simulink model "controlScheme_height"  (R2019b)
settings: Solver=FixedStepDiscrete  StartTime=0.0  StopTime=Inf  FixedStep=1/30  RelTol=1e-3
InitFcn:
  | tb = twinbeam('147.32.86.177', 30000);
  | gen = generator('147.32.86.177', 30001);
  | img = tb.get();
  | f = figure(25)
  | imshow(img);
  | [x_t, y_t] = ginput(1);
  | 
  | tb.tracker_init([y_t, x_t]);
  | 
  | 
  | delete(tb)
  | delete(gen)
  | pause(4)
  | close(f)
model workspace (MAT data in the model file):
  NumberOfBeads = Simulink.Parameter
  NumberOfBeads.Value = 1
  NumberOfBeads.DataType = 'auto'
  NumberOfBeads.Dimensions = [1 1]
undefined symbols (not defined in the file): DiscIntNeverNeededParam, H, Joystick, Standard_Devices, TCP_Protocol
libraries: sldrtlib x5, simulink x1
settings Model: SimulationMode=accelerator  EnablePacing=on  ParameterArgumentNames=NumberOfBeads  OrderedModelArguments=off  Creator=marti  LastModifiedBy=marti
settings SolverCC: MinimalZcImpactIntegration=on
settings DebuggingCC: ReadBeforeWriteMsg=DisableAll  WriteAfterWriteMsg=DisableAll  WriteAfterReadMsg=DisableAll  MultiTaskDSMMsg=none
settings ModelReferenceCC: UpdateModelReferenceTargets=IfOutOfDate
settings SFSimCC: SFSimEcho=off
settings RTWCC: Description=Simulink Desktop Real-Time  SystemTargetFile=sldrt.tlc  TemplateMakefile=sldrt.tmf  RTWCompilerOptimization=on
settings CodeAppCC: MaxIdLength=95
settings SimulinkDesktopRealTimeCC: TargetPreCompLibLocation=C:\Program Files\MATLAB\R2020a\toolbox\sldrt\lib\win64

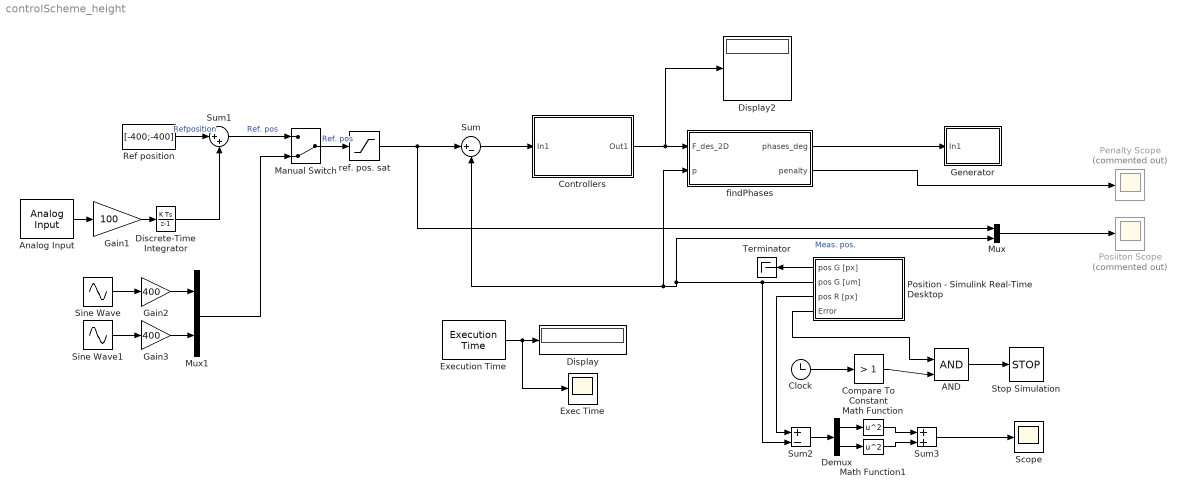
== system controlScheme_height ==
  AND : Logic  IconShape=distinctive  AllPortsSameDT=off  OutDataTypeStr=boolean
  Analog Input : sldrtlib/Analog Input  SampleTime=0.1  MaxMissedTicks=10  ShowMissedTicks=off  YieldWhenWaiting=off  DrvName=Standard_Devices/Joystick  DrvAddress=1  DrvOptions=zeros(1,0)  Channels=[1:2]  RangeMode=1  VoltRange=1  DataType=1
      settings: AttributesFormatString=Joystick [1]
  Clock : Clock
  Compare To Constant : simulink/Logic and Bit Operations/Compare To Constant  relop=>  const=1  OutDataTypeStr=boolean
  Controllers : Subsystem  mask{P_const=300e-14, F_max=30e-11}
      mask prompts: P_const "P constant"; F_max "F max"
  Demux : Demux  Outputs=2
  Discrete-Time Integrator : DiscreteIntegrator  gainval=1  SampleTime=-1  ICPrevOutput=DiscIntNeverNeededParam  ICPrevScaledInput=DiscIntNeverNeededParam
  Display : Display
  Display2 : Display
  Exec Time : Scope
  Execution Time : sldrtlib/Target Profiling/Execution Time  ShowTaskTimes=off
      settings: SourceProductBaseCode=WT
  Gain1 : Gain  Gain=100
  Gain2 : Gain  Gain=400
  Gain3 : Gain  Gain=400
  Generator : Subsystem
  Manual Switch : ManualSwitch  CurrentSetting=0
  Math Function : Math  Operator=square  SaturateOnIntegerOverflow=on
  Math Function1 : Math  Operator=square  SaturateOnIntegerOverflow=on
  Mux : Mux  Inputs=2
  Mux1 : Mux  Inputs=2
  Penalty Scope : Scope  Commented=on
  Posiiton Scope : Scope  Commented=on
  Position - Simulink Real-Time Desktop : Subsystem  VariantControl=(default)
  Ref position : Constant  Value=[-400;-400]
  Scope : Scope
  Sine Wave : Sin  Frequency=2*pi/40  SampleTime=0
  Sine Wave1 : Sin  Frequency=2*pi/20  Phase=-pi  SampleTime=0
  Stop Simulation : Stop
  Sum : Sum  Inputs=|+-
  Sum1 : Sum  Inputs=|++
  Sum2 : Sum  Inputs=+-
  Sum3 : Sum
  Terminator : Terminator
  findPhases : MATLAB Function  TreatAsAtomicUnit=on
  ref. pos. sat : Saturate  UpperLimit=600  LowerLimit=-600
  wires:
  Manual Switch/1 -> ref. pos. sat/1  "Ref. pos"
  Sum/1 -> Controllers/1(In1)
  Controllers/1(Out1) -> findPhases/1(F_des_2D), Display2/1
  Position - Simulink Real-Time Desktop/2(pos G [um]) -> Sum2/2, findPhases/2(p), Sum/2, Mux/2  "Meas. pos."
  Execution Time/1 -> Exec Time/1, Display/1
  findPhases/1(phases_deg) -> Generator/1(In1)
  findPhases/2(penalty) -> Penalty Scope/1
  AND/1 -> Stop Simulation/1
  Clock/1 -> Compare To Constant/1
  Compare To Constant/1 -> AND/2
  Position - Simulink Real-Time Desktop/4(Error) -> AND/1
  Mux/1 -> Posiiton Scope/1
  Analog Input/1 -> Gain1/1
  Ref position/1 -> Sum1/1  "Refposition"
  Discrete-Time Integrator/1 -> Sum1/2
  Gain1/1 -> Discrete-Time Integrator/1
  Sum1/1 -> Manual Switch/1  "Ref. pos"
  Sine Wave/1 -> Gain2/1
  Sine Wave1/1 -> Gain3/1
  Gain2/1 -> Mux1/1
  Gain3/1 -> Mux1/2
  Mux1/1 -> Manual Switch/2
  Position - Simulink Real-Time Desktop/1(pos G [px]) -> Terminator/1
  ref. pos. sat/1 -> Sum/1, Mux/1
  Position - Simulink Real-Time Desktop/3(pos R [px]) -> Sum2/1
  Sum2/1 -> Demux/1
  Demux/1 -> Math Function/1
  Demux/2 -> Math Function1/1
  Math Function/1 -> Sum3/1
  Math Function1/1 -> Sum3/2
  Sum3/1 -> Scope/1

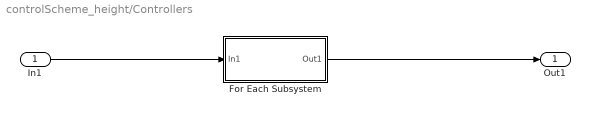
== system controlScheme_height/Controllers ==
  In1 : Inport
  For Each Subsystem : Subsystem  TreatAsAtomicUnit=on
  Out1 : Outport
  wires:
  In1/1 -> For Each Subsystem/1(In1)
  For Each Subsystem/1(Out1) -> Out1/1

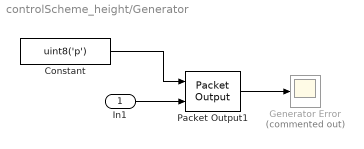
== system controlScheme_height/Generator ==
  In1 : Inport
  Constant : Constant  Value=uint8('p')
  Generator Error : Scope  Commented=on
  Packet Output1 : sldrtlib/Packet Output  SampleTime=1/30  MaxMissedTicks=20  ShowMissedTicks=off  YieldWhenWaiting=off  DrvName=Standard_Devices/TCP_Protocol  DrvAddress=30001  DrvOptions=[0 30001 49 52 55 46 51 50 46 56 54 46 49 55 55 0 0 0 0 0 0 0 0 0 0 0 0 0 0 0 0 0 0 0 0 0 0 0 0 0 0 0 0 0 0 0 0 0 0 0 0 0 0 0 0 0 0 0 0 0 0 0 0 0 0 0 0 0 0 0 0 0 0 0 0 0 0 0 0 0 0 0 0 0 0 0 0 0 0 0 0 0 0 0 0 0 0 0 0 0 0 0 0 0 0 0 0 0 0 0 0 0 0 0 0 0 0 0 0 0 0 0 0 0 0 0 0 0 0 0 0 0 0 0 0 0 0 0 0 0 0 0 0 0 0 0 0 0 0 0 0 0 0 0 0 0 0 0 0 0 0 0 0 0 0 0 0 0 0 0 0 0 0 0 0 0 0 0 0 0 0 0 0 0 0 0 0 0 0 0 0 0 0 0 0 0 0 0 0 0 0 0 0 0 0 0 0 0 0 0 0 0 0 0 0 0 0 0 0 0 0 0 0 0 0 0 0 0 0 0 0 0 0 0 0 0 0 0 0 0 0 0 0 0 0 0 0 0 0 0 0 0 0 0 0 0]  PacketSize=56*2+1  DataTypes={'uint8', '56*uint16'}  ShowReady=off  ShowError=on  PacketID=1  ByteOrder=1  InitialValue=[]  FinalValue=[]
      settings: AttributesFormatString=TCP Protocol [30001]
  wires:
  In1/1 -> Packet Output1/2
  Packet Output1/1 -> Generator Error/1
  Constant/1 -> Packet Output1/1

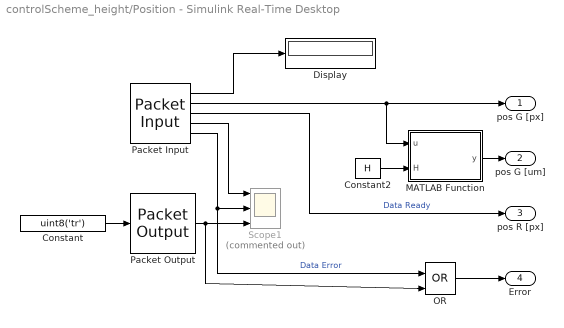
== system controlScheme_height/Position - Simulink Real-Time Desktop ==
  Constant : Constant  Value=uint8('tr')  OutDataTypeStr=uint8  SampleTime=-1
  Constant2 : Constant  Value=H
  Display : Display
      settings: Format=decimal (Stored Integer)
  MATLAB Function : MATLAB Function  TreatAsAtomicUnit=on
  OR : Logic  Operator=OR  IconShape=distinctive  AllPortsSameDT=off  OutDataTypeStr=boolean
  Packet Input : sldrtlib/Packet Input  SampleTime=1/30  MaxMissedTicks=20  ShowMissedTicks=off  YieldWhenWaiting=off  DrvName=Standard_Devices/TCP_Protocol  DrvAddress=30000  DrvOptions=[0 30000 49 52 55 46 51 50 46 56 54 46 49 55 55 0 0 0 0 0 0 0 0 0 0 0 0 0 0 0 0 0 0 0 0 0 0 0 0 0 0 0 0 0 0 0 0 0 0 0 0 0 0 0 0 0 0 0 0 0 0 0 0 0 0 0 0 0 0 0 0 0 0 0 0 0 0 0 0 0 0 0 0 0 0 0 0 0 0 0 0 0 0 0 0 0 0 0 0 0 0 0 0 0 0 0 0 0 0 0 0 0 0 0 0 0 0 0 0 0 0 0 0 0 0 0 0 0 0 0 0 0 0 0 0 0 0 0 0 0 0 0 0 0 0 0 0 0 0 0 0 0 0 0 0 0 0 0 0 0 0 0 0 0 0 0 0 0 0 0 0 0 0 0 0 0 0 0 0 0 0 0 0 0 0 0 0 0 0 0 0 0 0 0 0 0 0 0 0 0 0 0 0 0 0 0 0 0 0 0 0 0 0 0 0 0 0 0 0 0 0 0 0 0 0 0 0 0 0 0 0 0 0 0 0 0 0 0 0 0 0 0 0 0 0 0 0 0 0 0 0 0 0 0 0 0]  PacketSize=4+4+4  DataTypes={'uint32', '2*uint16', '2*uint16'}  ShowReady=on  ShowError=on  PacketID=1  ByteOrder=1  ShowTimestamp=off
      settings: AttributesFormatString=TCP Protocol [30000]
  Packet Output : sldrtlib/Packet Output  SampleTime=1/30  MaxMissedTicks=20  ShowMissedTicks=off  YieldWhenWaiting=off  DrvName=Standard_Devices/TCP_Protocol  DrvAddress=30000  DrvOptions=[0 30000 49 52 55 46 51 50 46 56 54 46 49 55 55 0 0 0 0 0 0 0 0 0 0 0 0 0 0 0 0 0 0 0 0 0 0 0 0 0 0 0 0 0 0 0 0 0 0 0 0 0 0 0 0 0 0 0 0 0 0 0 0 0 0 0 0 0 0 0 0 0 0 0 0 0 0 0 0 0 0 0 0 0 0 0 0 0 0 0 0 0 0 0 0 0 0 0 0 0 0 0 0 0 0 0 0 0 0 0 0 0 0 0 0 0 0 0 0 0 0 0 0 0 0 0 0 0 0 0 0 0 0 0 0 0 0 0 0 0 0 0 0 0 0 0 0 0 0 0 0 0 0 0 0 0 0 0 0 0 0 0 0 0 0 0 0 0 0 0 0 0 0 0 0 0 0 0 0 0 0 0 0 0 0 0 0 0 0 0 0 0 0 0 0 0 0 0 0 0 0 0 0 0 0 0 0 0 0 0 0 0 0 0 0 0 0 0 0 0 0 0 0 0 0 0 0 0 0 0 0 0 0 0 0 0 0 0 0 0 0 0 0 0 0 0 0 0 0 0 0 0 0 0 0 0]  PacketSize=2  DataTypes='2*uint8'  ShowReady=off  ShowError=on  PacketID=1  ByteOrder=1  InitialValue=[]  FinalValue=[]
      settings: AttributesFormatString=TCP Protocol [30000]
  Scope1 : Scope  Commented=on  NumInputPorts=3
  pos G [px] : Outport
  pos G [um] : Outport  Port=2  Unit=um
  pos R [px] : Outport  Port=3
  Error : Outport  Port=4
  wires:
  Packet Input/5 -> OR/1, Scope1/2  "Data Error"
  Packet Input/2 -> MATLAB Function/1(u), pos G [px]/1
  Packet Input/1 -> Display/1
  Packet Input/4 -> Scope1/1
  Constant/1 -> Packet Output/1
  Constant2/1 -> MATLAB Function/2(H)
  MATLAB Function/1(y) -> pos G [um]/1
  OR/1 -> Error/1
  Packet Output/1 -> Scope1/3, OR/2
  Packet Input/3 -> pos R [px]/1  "Data Ready"

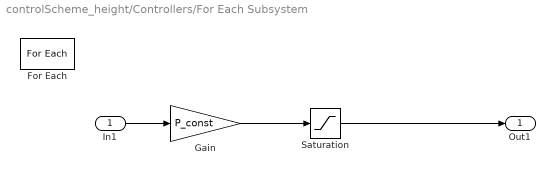
== system controlScheme_height/Controllers/For Each Subsystem ==
  In1 : Inport  Partition=on  PartitionDimension=1  PartitionWidth=2  PartitionOffset=0
  For Each : ForEach  DisableCoverage=on
  Gain : Gain  Gain=P_const
  Saturation : Saturate  UpperLimit=F_max  LowerLimit=-F_max
  Out1 : Outport  ConcatenationDimension=1
  wires:
  In1/1 -> Gain/1
  Gain/1 -> Saturation/1
  Saturation/1 -> Out1/1

== matlab function controlScheme_height/findPhases ==
  data: F_des_2D input; p input; phases_deg output; penalty output
function [phases_deg, penalty] = fcn(F_des_2D, p)
ParticleRadisu = 25e-6;
ParticleDensity = 1.05e3;
MediumDensity = 0.998e3;
g = 9.81373; % m/s^2
F_z = -4/3*pi*ParticleRadisu^3*(MediumDensity-ParticleDensity)*g;
F_des = [0;0;F_z];
p_z = 130e-6;
position = [0;0;p_z];

F_des(1:2) = F_des_2D;
position(1:2) = p*1e-6;
[phases_rad, penalty] = findPhasesFoGivenF(position, F_des);
phases_deg = rad2deg(phases_rad);
phases_deg = round(mod(phases_deg, 360));

== matlab function controlScheme_height/Position - Simulink Real-Time Desktop/MATLAB Function ==
  data: u input; y output; H input
function y = fcn(u, H)
tmp = H*[double(u(2));double(u(1));1];
y = [tmp(1)/tmp(3); tmp(2)/tmp(3)];
